simulink model "MRAC_IU"  (R2021a)
settings: Solver=ode23  StartTime=0.0  StopTime=150  RelTol=1e-6  AbsTol=1e-6
settings Model: Creator=valerio  LastModifiedBy=simon

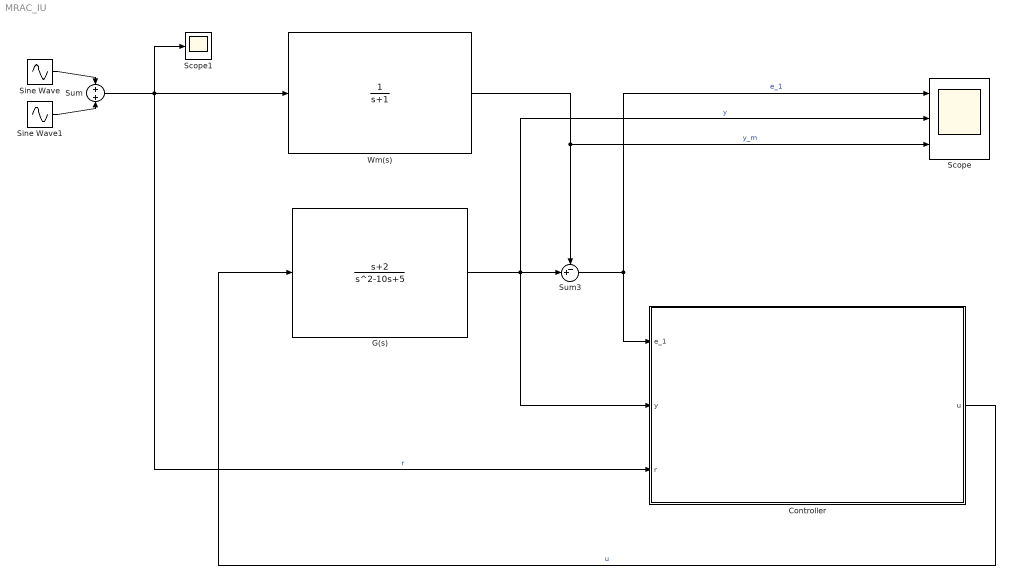
== system MRAC_IU ==
  Controller : Subsystem
  G(s) : TransferFcn  Numerator=[1 2]  Denominator=[1 -10 5]
  Scope : Scope  NumInputPorts=3
  Scope1 : Scope
  Sine Wave : Sin  Frequency=2  SampleTime=0
  Sine Wave1 : Sin  Frequency=0.5  SampleTime=0
  Sum : Sum
  Sum3 : Sum  Inputs=-+|
  Wm(s) : TransferFcn  Denominator=[1 1]
  wires:
  Sine Wave/1 -> Sum/1
  Sine Wave1/1 -> Sum/2
  Sum/1 -> Scope1/1, Wm(s)/1, Controller/3(r)  "r"
  G(s)/1 -> Controller/2(y), Sum3/2, Scope/2  "y"
  Wm(s)/1 -> Sum3/1, Scope/3  "y_m"
  Sum3/1 -> Scope/1, Controller/1(e_1)  "e_1"
  Controller/1(u) -> G(s)/1  "u"

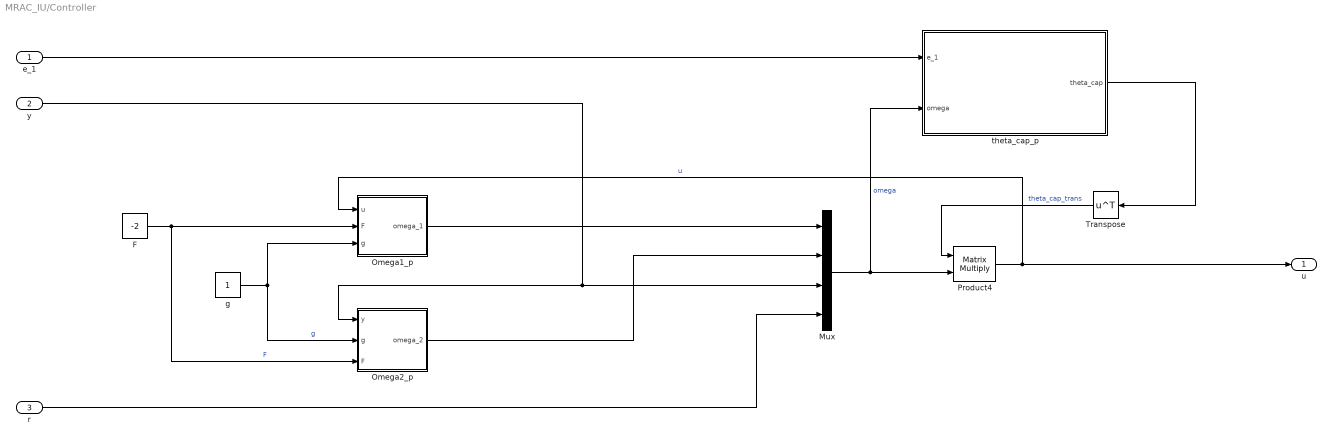
== system MRAC_IU/Controller ==
  e_1 : Inport
  y : Inport  Port=2
  r : Inport  Port=3
  F : Constant  Value=-2
  Mux : Mux
  Omega1_p : Subsystem
  Omega2_p : Subsystem
  Product4 : Product  Multiplication=Matrix(*)
  Transpose : Math  Operator=transpose  SaturateOnIntegerOverflow=on
  g : Constant
  theta_cap_p : Subsystem
  u : Outport
  wires:
  Transpose/1 -> Product4/1  "theta_cap_trans"
  Omega1_p/1(omega_1) -> Mux/1
  g/1 -> Omega2_p/2(g), Omega1_p/3(g)  "g"
  Mux/1 -> Product4/2, theta_cap_p/2(omega)  "omega"
  Product4/1 -> u/1, Omega1_p/1(u)  "u"
  F/1 -> Omega1_p/2(F), Omega2_p/3(F)  "F"
  r/1 -> Mux/4
  y/1 -> Mux/3, Omega2_p/1(y)
  Omega2_p/1(omega_2) -> Mux/2
  theta_cap_p/1(theta_cap) -> Transpose/1
  e_1/1 -> theta_cap_p/1(e_1)

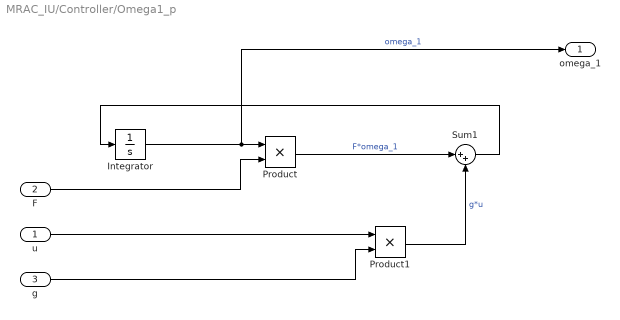
== system MRAC_IU/Controller/Omega1_p ==
  u : Inport
  F : Inport  Port=2
  g : Inport  Port=3
  Integrator : Integrator
  Product : Product
  Product1 : Product
  Sum1 : Sum  Inputs=|++
  omega_1 : Outport
  wires:
  u/1 -> Product1/1
  Product/1 -> Sum1/1  "F*omega_1"
  F/1 -> Product/2
  g/1 -> Product1/2
  Product1/1 -> Sum1/2  "g*u"
  Integrator/1 -> omega_1/1, Product/1  "omega_1"
  Sum1/1 -> Integrator/1

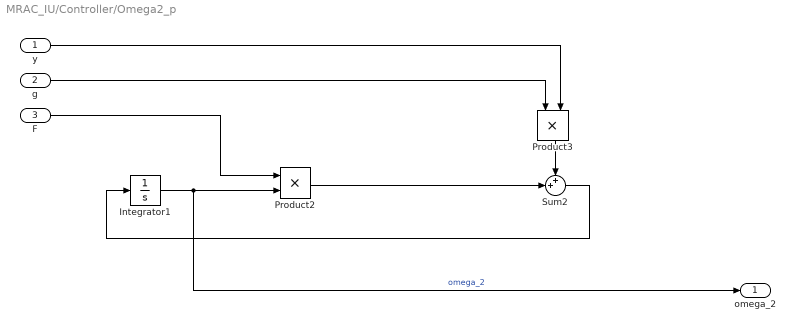
== system MRAC_IU/Controller/Omega2_p ==
  y : Inport
  g : Inport  Port=2
  F : Inport  Port=3
  Integrator1 : Integrator
  Product2 : Product
  Product3 : Product
  Sum2 : Sum  Inputs=++|
  omega_2 : Outport
  wires:
  g/1 -> Product3/1
  Product2/1 -> Sum2/2
  y/1 -> Product3/2
  Integrator1/1 -> Product2/2, omega_2/1  "omega_2"
  Product3/1 -> Sum2/1
  F/1 -> Product2/1
  Sum2/1 -> Integrator1/1

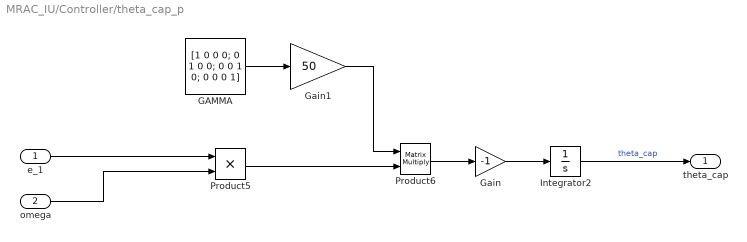
== system MRAC_IU/Controller/theta_cap_p ==
  e_1 : Inport
  omega : Inport  Port=2
  GAMMA : Constant  Value=[1 0 0 0; 0 1 0 0; 0 0 1 0; 0 0 0 1]
  Gain : Gain  Gain=-1
  Gain1 : Gain  Gain=50
  Integrator2 : Integrator
  Product5 : Product
  Product6 : Product  Multiplication=Matrix(*)
  theta_cap : Outport
  wires:
  Integrator2/1 -> theta_cap/1  "theta_cap"
  Product6/1 -> Gain/1
  Product5/1 -> Product6/2
  GAMMA/1 -> Gain1/1
  Gain1/1 -> Product6/1
  e_1/1 -> Product5/1
  omega/1 -> Product5/2
  Gain/1 -> Integrator2/1
